simulink model "tutorial38_bus"  (R2025a)
settings: Solver=VariableStepAuto  StartTime=0.0  StopTime=10.0  RelTol=1e-3
settings Model: Creator=xing2  LastModifiedBy=xing2

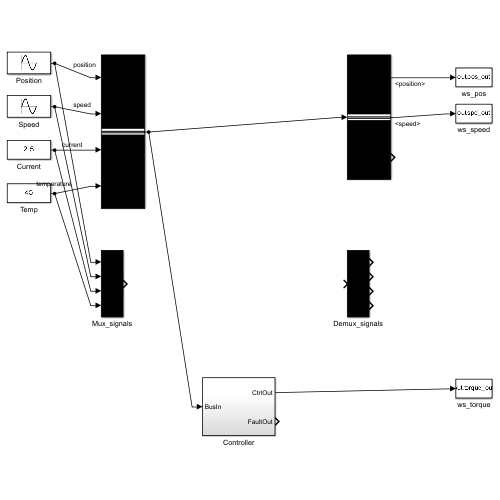
[thumbnail: Simulink's stored preview of the top-level diagram]
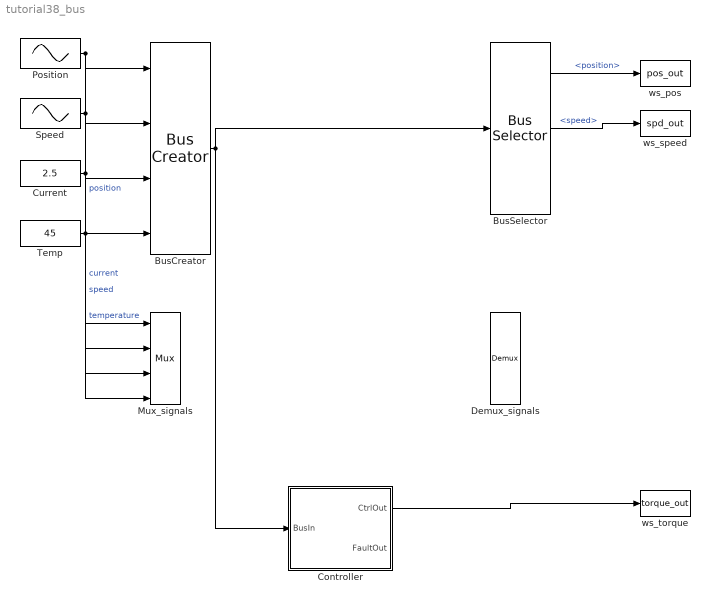
== system tutorial38_bus ==
  BusCreator : BusCreator  Inputs=4
  BusSelector : BusSelector  OutputSignals=position,speed,temperature
  Controller : Subsystem
  Current : Constant  Value=2.5
  Demux_signals : Demux
  Mux_signals : Mux
  Position : Sin  Frequency=0.5  SampleTime=0
  Speed : Sin  Amplitude=3  Frequency=0.5  Phase=pi/2  SampleTime=0
  Temp : Constant  Value=45
  ws_pos : ToWorkspace  VariableName=pos_out  SaveFormat=Timeseries  SampleTime=-1
  ws_speed : ToWorkspace  VariableName=spd_out  SaveFormat=Timeseries  SampleTime=-1
  ws_torque : ToWorkspace  VariableName=torque_out  SaveFormat=Timeseries  SampleTime=-1
  wires:
  Position/1 -> BusCreator/1, Mux_signals/1  "position"
  Speed/1 -> BusCreator/2, Mux_signals/2  "speed"
  Current/1 -> BusCreator/3, Mux_signals/3  "current"
  Temp/1 -> BusCreator/4, Mux_signals/4  "temperature"
  BusCreator/1 -> BusSelector/1, Controller/1(BusIn)
  BusSelector/1 -> ws_pos/1  "<position>"
  BusSelector/2 -> ws_speed/1  "<speed>"
  Controller/1(CtrlOut) -> ws_torque/1

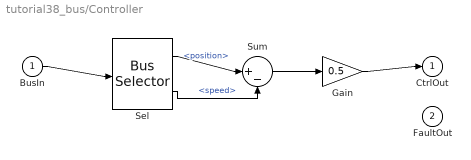
== system tutorial38_bus/Controller ==
  BusIn : Inport
  Gain : Gain  Gain=0.5
  Sel : BusSelector  OutputSignals=position,speed
  Sum : Sum  Inputs=|+-
  CtrlOut : Outport
  FaultOut : Outport  Port=2
  wires:
  BusIn/1 -> Sel/1
  Sel/1 -> Sum/1  "<position>"
  Sel/2 -> Sum/2  "<speed>"
  Sum/1 -> Gain/1
  Gain/1 -> CtrlOut/1
